simulink model "PropGlycAdjustedARNew1"  (R2019a)
settings: Solver=FixedStepAuto  StartTime=0.0  StopTime=4000  FixedStep=0.1  RelTol=1e-3
values from neighbouring files (symbols this model uses):
  As = pi*r^2    (= 1.89569430983)    [GlycolCSTRparam.m]
  Atank = 6^2*pi()    [GlycolCSTRparam.m]
  Cpa = 35    [GlycolCSTRparam.m]
  Cpb = 18    [GlycolCSTRparam.m]
  Cpc = 46    [GlycolCSTRparam.m]
  Cpm = 19.5    [GlycolCSTRparam.m]
  Cpw = 18    [GlycolCSTRparam.m]
  den = 2.6729    [GlycolCSTRparam.m]
  dh = -36000    [GlycolCSTRparam.m]
  EA = 32400    [GlycolCSTRparam.m]
  Fao = 80    [GlycolCSTRparam.m]
  Fbo = 1000    [GlycolCSTRparam.m]    (also in groundtruth.m)
  Fmo = 100    [GlycolCSTRparam.m]    (also in groundtruth.m)
  htankmax = Vtankmax/Atank    [GlycolCSTRparam.m]
  Hvap = 18279    [GlycolCSTRparam.m]
  Kla = 0    [GlycolCSTRparam.m]
  ko = 16.96e12    (= 16960000000000)    [GlycolCSTRparam.m]
  KT = -10    [GlycolCSTRparam.m]
  Ktank = -1000    [GlycolCSTRparam.m]
  KTank1 = -20    [GlycolCSTRparam.m]
  mc = 1000    [GlycolCSTRparam.m]
  pa = 0.923    [GlycolCSTRparam.m]
  pb = 3.45    [GlycolCSTRparam.m]
  pm = 1.54    [GlycolCSTRparam.m]
  R = 1.987    [GlycolCSTRparam.m]
  RandomMatrix = RandomSetTest    [FinalThesis.m]
  tauT = 2    [GlycolCSTRparam.m]
  tauTank = 0.2    [GlycolCSTRparam.m]
  Tc = 60    [GlycolCSTRparam.m]    (also in groundtruth.m)
  To = 75    [GlycolCSTRparam.m]    (also in groundtruth.m)
  UA = 16000    [GlycolCSTRparam.m]
  V = (1/7.484)*500    (= 66.8091929449)    [GlycolCSTRparam.m]    (also in PCmodel.m = fliplr(V); isstat.m = D(:,j)'; isstatshift.m = D(:,j)')
  Vo = Fao/0.923+Fbo/3.45+Fmo/1.54    (= 441.46402689)    [GlycolCSTRparam.m]
undefined symbols (not defined in the file or in its folder): Tb
settings Model: Creator=19184956  LastModifiedBy=19184956

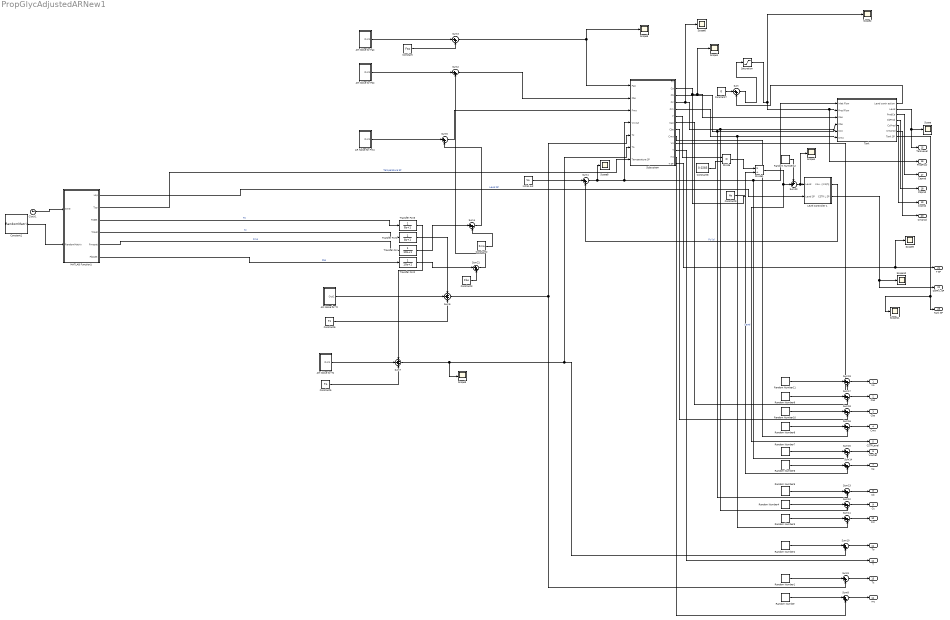
== system PropGlycAdjustedARNew1 ==
  AR Noise for Fao : Subsystem
  AR Noise for Fbo : Subsystem
  AR Noise for Fmo : Subsystem
  AR Noise for Tc : Subsystem
  AR Noise for To : Subsystem
  Clock1 : Clock
  Constant : Constant  Value=Fao
  Constant1 : Constant  Value=RandomMatrix  VectorParams1D=off  SampleTime=-1
  Constant2 : Constant  Value=Fmo
  Constant3 : Constant  Value=Fbo
  Constant5 : Constant  Value=To
  Constant6 : Constant  Value=Tc
  Constant7 : Constant  Value=0
  Constant8 : Constant  Value=0.0283
  Constant9 : Constant  Value=As
  Divide : Product  Inputs=**
  Divide1 : Product  Inputs=*/
  Initial out : Constant  Value=Vo
  Level Controller 1 : Subsystem
  MATLAB Function1 : MATLAB Function  TreatAsAtomicUnit=on
  Random Number{,1..2,7,11} (5 alike) : RandomNumber  Variance=0.5  SampleTime=0.1
  Random Number{3..6,8..10} (7 alike) : RandomNumber  Variance=0.0000025  SampleTime=0.1
  Random Number12 : RandomNumber  Variance=0.0002  SampleTime=0.1
  Saturation : Saturate  UpperLimit=inf  LowerLimit=0
  Scope{,1..6,8..11} (11 alike) : Scope
  Subsystem : Subsystem
  Sum{,1..5,8..19,21} (19 alike) : Sum  Inputs=|++
  Sum20 : Sum  Inputs=++|
  Sum6 : Sum  Inputs=+++
  Sum7 : Sum  Inputs=+++
  Tank : Subsystem
  Transfer Fcn : TransferFcn  Denominator=[10 1]
  Transfer Fcn1 : TransferFcn  Denominator=[8 1]
  Transfer Fcn2 : TransferFcn  Denominator=[10 1]
  Transfer Fcn3 : TransferFcn  Denominator=[8 1]
  Vo : Outport
  Cao : Outport  Port=2
  Cbo : Outport  Port=3
  Cmo : Outport  Port=4
  CSTRLevel : Outport  Port=5
  Voutlet : Outport  Port=6
  Ca : Outport  Port=7
  Cb : Outport  Port=8
  Cc : Outport  Port=9
  Cm : Outport  Port=10
  To : Outport  Port=11
  T : Outport  Port=12
  Tc : Outport  Port=13
  mc : Outport  Port=14
  TankLevel : Outport  Port=15
  ProdFlow : Outport  Port=16
  Caprod : Outport  Port=17
  Cbprod : Outport  Port=18
  Ccprod : Outport  Port=19
  Cmprod : Outport  Port=20
  T SP : Outport  Port=21
  CSTR L SP : Outport  Port=22
  Tank SP : Outport  Port=23
  wires:
  Sum2/1 -> Subsystem/2(Fbo)
  Constant2/1 -> Sum4/2
  Initial out/1 -> Sum1/1
  Sum6/1 -> Subsystem/5(Tc), Sum9/2
  Sum7/1 -> Scope3/1, Sum10/2, Subsystem/6(To)
  Subsystem/2(Ca) -> Sum14/2, Tank/3(Cao), Scope1/1
  Subsystem/3(Cb) -> Tank/4(Cbo), Sum13/2
  Subsystem/4(Cc) -> Scope6/1, Tank/5(Cco), Sum12/2
  Subsystem/5(Cm) -> Tank/6(Cmo), Sum11/2
  Sum/1 -> Saturation/1
  Tank/2(Level) -> TankLevel/1, Scope/1
  Constant7/1 -> Sum/1
  Tank/1(Level contr action) -> Sum/2
  Subsystem/6(V) -> Divide/1
  Constant8/1 -> Divide/2
  Divide/1 -> Divide1/1
  Constant9/1 -> Divide1/2
  Divide1/1 -> CSTRLevel/1, Sum20/2  "Level"
  Level Controller 1/1(Vout'(s) [m3/h]) -> Sum1/2  "Fc'(s)"
  Sum1/1 -> Scope8/1, Tank/1(Inlet Flow), Sum15/2, Subsystem/4(Vo out)
  Saturation/1 -> Scope2/1, ProdFlow/1, Tank/2(Prod Flow)
  Subsystem/10(Vo) -> Sum19/2
  Subsystem/7(Cao) -> Sum17/2
  Subsystem/8(Cbo) -> Sum18/2
  Subsystem/9(Cmo) -> Sum16/2
  Subsystem/11(T) -> T/1
  Subsystem/12(mc) -> Sum8/2
  Tank/3(ProdCa) -> Caprod/1
  Tank/4(CbProd) -> Cbprod/1
  Tank/5(CcProd) -> Ccprod/1
  Tank/6(Cmprod) -> Cmprod/1
  Subsystem/13(T SP) -> Scope9/1, T SP/1
  Level Controller 1/2(CSTR L SP) -> CSTR L SP/1, Scope10/1
  Tank/7("Tank SP ") -> Scope11/1, Tank SP/1
  Sum3/1 -> Subsystem/1(Fao), Scope5/1
  MATLAB Function1/2(Tsp) -> Subsystem/7(Temperature SP)  "Temperature SP"
  MATLAB Function1/1(Lsp) -> Level Controller 1/2(Level SP)  "Level SP"
  Transfer Fcn/1 -> Sum4/1
  Constant/1 -> Sum3/2
  Sum5/1 -> Subsystem/3(Fmo)
  AR Noise for Fao/1(Out1) -> Sum3/1
  AR Noise for Fbo/1(Out1) -> Sum2/1
  Sum4/1 -> Sum5/2
  AR Noise for Fmo/1(Out1) -> Sum5/1
  Constant6/1 -> Sum6/3
  Random Number/1 -> Sum8/1
  Sum8/1 -> mc/1
  Sum9/1 -> Tc/1
  Random Number1/1 -> Sum9/1
  Random Number2/1 -> Sum10/1
  Sum10/1 -> To/1
  Random Number3/1 -> Sum11/1
  Sum11/1 -> Cm/1
  Random Number4/1 -> Sum12/1
  Random Number5/1 -> Sum13/1
  Random Number6/1 -> Sum14/1
  Sum12/1 -> Cc/1
  Sum13/1 -> Cb/1
  Sum14/1 -> Ca/1
  Random Number7/1 -> Sum15/1
  Sum15/1 -> Voutlet/1
  Sum16/1 -> Cmo/1
  Random Number8/1 -> Sum16/1
  Sum17/1 -> Cao/1
  Random Number9/1 -> Sum17/1
  Sum18/1 -> Cbo/1
  Random Number10/1 -> Sum18/1
  Sum19/1 -> Vo/1
  Random Number11/1 -> Sum19/1
  Sum20/1 -> Scope4/1, Level Controller 1/1(Level)
  Random Number12/1 -> Sum20/1
  Transfer Fcn1/1 -> Sum6/1
  AR Noise for Tc/1(Out1) -> Sum6/2
  Transfer Fcn2/1 -> Sum21/1
  Constant3/1 -> Sum21/2
  Sum21/1 -> Sum2/2
  Transfer Fcn3/1 -> Sum7/1
  AR Noise for To/1(Out1) -> Sum7/2
  Constant5/1 -> Sum7/3
  Constant1/1 -> MATLAB Function1/2(RandomMatrix)
  Clock1/1 -> MATLAB Function1/1(time)
  MATLAB Function1/4(Tcset) -> Transfer Fcn1/1  "Tc"
  MATLAB Function1/6(Fboset) -> Transfer Fcn2/1  "Fbo"
  MATLAB Function1/3(ToSet) -> Transfer Fcn3/1  "To"
  MATLAB Function1/5(Fmoset) -> Transfer Fcn/1  "Fmo"

== system PropGlycAdjustedARNew1/AR Noise for Fao ==
  Clock1 : Clock
  Gain : Gain  Gain=0.7
  Random Number : RandomNumber  Variance=0.005  SampleTime=2
  Random Number1 : RandomNumber  Variance=0.005  SampleTime=0.5
  Sum2 : Sum  Inputs=|++
  Switch : Switch  Criteria=u2 > Threshold  Threshold=10
  Transport Delay : TransportDelay  DelayTime=2
  Out1 : Outport
  wires:
  Random Number1/1 -> Switch/3
  Gain/1 -> Sum2/1
  Sum2/1 -> Out1/1, Transport Delay/1
  Random Number/1 -> Switch/1
  Switch/1 -> Sum2/2
  Clock1/1 -> Switch/2
  Transport Delay/1 -> Gain/1

== system PropGlycAdjustedARNew1/AR Noise for Fbo ==
  Clock1 : Clock
  Gain : Gain  Gain=0.7
  Random Number : RandomNumber  Variance=0.005  SampleTime=2
  Random Number1 : RandomNumber  Variance=0.005  SampleTime=0.5
  Scope : Scope
  Sum2 : Sum  Inputs=|++
  Switch : Switch  Criteria=u2 > Threshold  Threshold=10
  Transport Delay : TransportDelay  DelayTime=2
  Out1 : Outport
  wires:
  Random Number1/1 -> Switch/3
  Gain/1 -> Sum2/1
  Sum2/1 -> Scope/1, Out1/1, Transport Delay/1
  Random Number/1 -> Switch/1
  Switch/1 -> Sum2/2
  Clock1/1 -> Switch/2
  Transport Delay/1 -> Gain/1

== system PropGlycAdjustedARNew1/AR Noise for Fmo ==
  Clock1 : Clock
  Gain : Gain  Gain=0.7
  Random Number : RandomNumber  Variance=0.005  SampleTime=2
  Random Number1 : RandomNumber  Variance=0  SampleTime=0.5
  Sum2 : Sum  Inputs=|++
  Switch : Switch  Criteria=u2 > Threshold  Threshold=10
  Transport Delay : TransportDelay  DelayTime=2
  Out1 : Outport
  wires:
  Random Number1/1 -> Switch/3
  Gain/1 -> Sum2/1
  Sum2/1 -> Out1/1, Transport Delay/1
  Random Number/1 -> Switch/1
  Switch/1 -> Sum2/2
  Clock1/1 -> Switch/2
  Transport Delay/1 -> Gain/1

== system PropGlycAdjustedARNew1/AR Noise for Tc ==
  Clock1 : Clock
  Gain : Gain  Gain=0.7
  Random Number : RandomNumber  Variance=0.05  SampleTime=2
  Random Number1 : RandomNumber  Variance=0  SampleTime=0.5
  Sum2 : Sum  Inputs=|++
  Switch : Switch  Criteria=u2 > Threshold  Threshold=10
  Transport Delay : TransportDelay  DelayTime=2
  Out1 : Outport
  wires:
  Random Number1/1 -> Switch/3
  Gain/1 -> Sum2/1
  Sum2/1 -> Out1/1, Transport Delay/1
  Random Number/1 -> Switch/1
  Switch/1 -> Sum2/2
  Clock1/1 -> Switch/2
  Transport Delay/1 -> Gain/1

== system PropGlycAdjustedARNew1/AR Noise for To ==
  Clock1 : Clock
  Gain : Gain  Gain=0.7
  Random Number : RandomNumber  Variance=0.05  SampleTime=2
  Random Number1 : RandomNumber  Variance=0  SampleTime=0.5
  Sum2 : Sum  Inputs=|++
  Switch : Switch  Criteria=u2 > Threshold  Threshold=10
  Transport Delay : TransportDelay  DelayTime=2
  Out1 : Outport
  wires:
  Random Number1/1 -> Switch/3
  Gain/1 -> Sum2/1
  Sum2/1 -> Out1/1, Transport Delay/1
  Random Number/1 -> Switch/1
  Switch/1 -> Sum2/2
  Clock1/1 -> Switch/2
  Transport Delay/1 -> Gain/1

== system PropGlycAdjustedARNew1/Level Controller 1 ==
  Level : Inport
  Level SP : Inport  Port=2
  Constant1 : Constant  Value=0.98
  Gain5 : Gain  Gain=KTank1
  Gc1 : TransferFcn  Numerator=[tauTank 1]  Denominator=[tauTank 0]
  Scope : Scope
  Sum : Sum  Inputs=-+|
  Sum1 : Sum  Inputs=|-+
  Transfer Fcn : TransferFcn  Denominator=[4 1]
  Vout'(s) [m3/h] : Outport
  CSTR L SP : Outport  Port=2
  wires:
  Sum/1 -> Sum1/1  "T'(s)"
  Sum1/1 -> Gain5/1  "E1(s) [K]"
  Constant1/1 -> Sum/1
  Gc1/1 -> Scope/1, Vout'(s) [m3/h]/1  "Vout'(s) [m3/h]"
  Level SP/1 -> Transfer Fcn/1, CSTR L SP/1
  Gain5/1 -> Gc1/1
  Level/1 -> Sum/2
  Transfer Fcn/1 -> Sum1/2

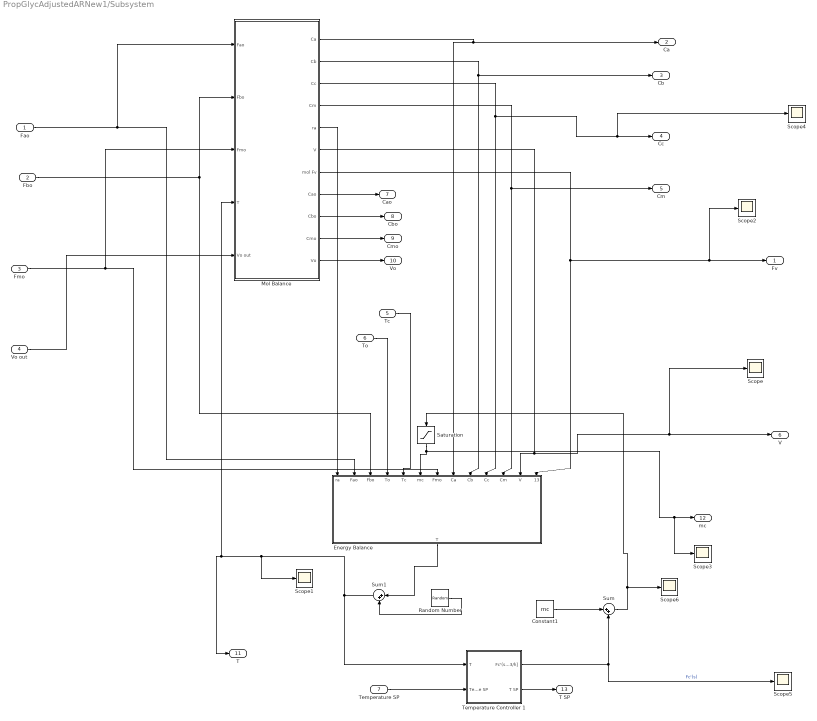
== system PropGlycAdjustedARNew1/Subsystem ==
  Fao : Inport
  Fbo : Inport  Port=2
  Fmo : Inport  Port=3
  Vo out : Inport  Port=4
  Tc : Inport  Port=5
  To : Inport  Port=6
  Temperature SP : Inport  Port=7
  Constant1 : Constant  Value=mc
  Energy Balance : Subsystem
  Mol Balance : Subsystem
  Random Number : RandomNumber  Variance=0.005  SampleTime=0.1
  Saturation : Saturate  UpperLimit=inf  LowerLimit=10
  Scope{,1..6} (7 alike) : Scope
  Sum : Sum  Inputs=|++
  Sum1 : Sum  Inputs=|++
  Temperature Controller 1 : Subsystem
  Fv : Outport
  Ca : Outport  Port=2
  Cb : Outport  Port=3
  Cc : Outport  Port=4
  Cm : Outport  Port=5
  V : Outport  Port=6
  Cao : Outport  Port=7
  Cbo : Outport  Port=8
  Cmo : Outport  Port=9
  Vo : Outport  Port=10
  T : Outport  Port=11
  mc : Outport  Port=12
  T SP : Outport  Port=13
  wires:
  Fmo/1 -> Energy Balance/7(Fmo), Mol Balance/3(Fmo)
  Tc/1 -> Energy Balance/5(Tc)
  Mol Balance/2(Cb) -> Energy Balance/9(Cb), Cb/1
  Mol Balance/4(Cm) -> Cm/1, Energy Balance/11(Cm)
  Mol Balance/7(mol Fv) -> Scope2/1, Fv/1, Energy Balance/13("Fv mol ")
  Mol Balance/3(Cc) -> Scope4/1, Cc/1, Energy Balance/10(Cc)
  Vo out/1 -> Mol Balance/5(Vo out)
  Mol Balance/5(ra) -> Energy Balance/1(ra)
  Fbo/1 -> Energy Balance/3(Fbo), Mol Balance/2(Fbo)
  To/1 -> Energy Balance/4(To)
  Fao/1 -> Energy Balance/2(Fao), Mol Balance/1(Fao)
  Mol Balance/1(Ca) -> Ca/1, Energy Balance/8(Ca)
  Mol Balance/6(V) -> Scope/1, V/1, Energy Balance/12(V)
  Temperature Controller 1/1(Fc'(s) [m3/h]) -> Scope5/1, Sum/2  "Fc'(s)"
  Constant1/1 -> Sum/1
  Sum/1 -> Scope6/1, Saturation/1
  Mol Balance/8(Cao) -> Cao/1
  Mol Balance/9(Cbo) -> Cbo/1
  Mol Balance/10(Cmo) -> Cmo/1
  Mol Balance/11(Vo) -> Vo/1
  Sum1/1 -> Scope1/1, T/1, Mol Balance/4(T), Temperature Controller 1/1(T)
  Temperature Controller 1/2(T SP) -> T SP/1
  Saturation/1 -> Scope3/1, mc/1, Energy Balance/6(mc)
  Temperature SP/1 -> Temperature Controller 1/2(Temperature SP)
  Random Number/1 -> Sum1/2
  Energy Balance/1(T) -> Sum1/1

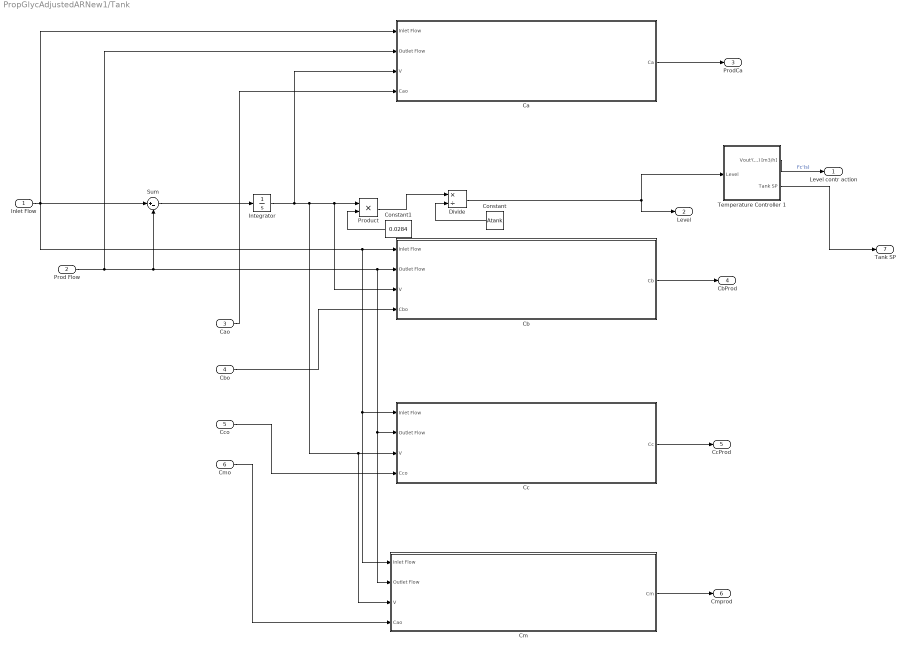
== system PropGlycAdjustedARNew1/Tank ==
  Inlet Flow : Inport
  Prod Flow : Inport  Port=2
  Cao : Inport  Port=3
  Cbo : Inport  Port=4
  Cco : Inport  Port=5
  Cmo : Inport  Port=6
  Ca : Subsystem
  Cb : Subsystem
  Cc : Subsystem
  Cm : Subsystem
  Constant : Constant  Value=Atank
  Constant1 : Constant  Value=0.0284
  Divide : Product  Inputs=*/
  Integrator : Integrator  InitialCondition=V*0.1  UpperSaturationLimit=V
  Product : Product
  Sum : Sum  Inputs=|+-
  Temperature Controller 1 : Subsystem
  Level contr action : Outport
  Level : Outport  Port=2
  ProdCa : Outport  Port=3
  CbProd : Outport  Port=4
  CcProd : Outport  Port=5
  Cmprod : Outport  Port=6
  "Tank SP " : Outport  Port=7
  wires:
  Integrator/1 -> Ca/3(V), Cm/3(V), Cc/3(V), Product/1, Cb/3(V)
  Sum/1 -> Integrator/1
  Inlet Flow/1 -> Ca/1(Inlet Flow), Cm/1(Inlet Flow), Cc/1(Inlet Flow), Cb/1(Inlet Flow), Sum/1
  Prod Flow/1 -> Ca/2(Outlet Flow), Cm/2(Outlet Flow), Cc/2(Outlet Flow), Cb/2(Outlet Flow), Sum/2
  Cao/1 -> Ca/4(Cao)
  Cbo/1 -> Cb/4(Cbo)
  Cco/1 -> Cc/4(Cco)
  Cmo/1 -> Cm/4(Cao)
  Constant/1 -> Divide/2
  Divide/1 -> Temperature Controller 1/1(Level), Level/1
  Temperature Controller 1/1(Vout'(s) [m3/h]) -> Level contr action/1  "Fc'(s)"
  Constant1/1 -> Product/2
  Product/1 -> Divide/1
  Ca/1(Ca) -> ProdCa/1
  Cb/1(Cb) -> CbProd/1
  Cc/1(Cc) -> CcProd/1
  Cm/1(Cm) -> Cmprod/1
  Temperature Controller 1/2(Tank SP) -> "Tank SP "/1

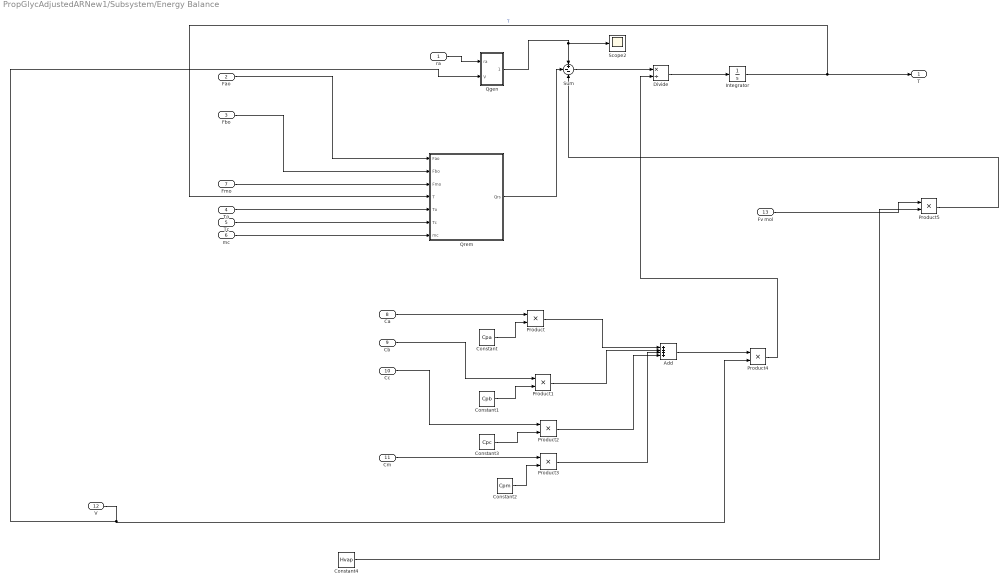
== system PropGlycAdjustedARNew1/Subsystem/Energy Balance ==
  ra : Inport
  Fao : Inport  Port=2
  Fbo : Inport  Port=3
  To : Inport  Port=4
  Tc : Inport  Port=5
  mc : Inport  Port=6
  Fmo : Inport  Port=7
  Ca : Inport  Port=8
  Cb : Inport  Port=9
  Cc : Inport  Port=10
  Cm : Inport  Port=11
  V : Inport  Port=12
  "Fv mol " : Inport  Port=13
  Add : Sum  Inputs=++++
  Constant : Constant  Value=Cpa
  Constant1 : Constant  Value=Cpb
  Constant2 : Constant  Value=Cpm
  Constant3 : Constant  Value=Cpc
  Constant4 : Constant  Value=Hvap
  Divide : Product  Inputs=*/
  Integrator : Integrator  InitialCondition=To  UpperSaturationLimit=Tb+0.5
  Product{,1..5} (6 alike) : Product
  Qgen : Subsystem
  Qrem : Subsystem
  Scope2 : Scope
  Sum : Sum  Inputs=+--
  T : Outport
  wires:
  Integrator/1 -> T/1, Qrem/4(T)  "T"
  ra/1 -> Qgen/1(ra)
  Qrem/1(Qrs) -> Sum/2
  Fao/1 -> Qrem/1(Fao)
  Fbo/1 -> Qrem/2(Fbo)
  To/1 -> Qrem/5(To)
  Tc/1 -> Qrem/6(Tc)
  mc/1 -> Qrem/7(mc)
  Fmo/1 -> Qrem/3(Fmo)
  Ca/1 -> Product/1
  Cb/1 -> Product1/1
  Cc/1 -> Product2/1
  Cm/1 -> Product3/1
  Constant/1 -> Product/2
  Constant1/1 -> Product1/2
  Constant3/1 -> Product2/2
  Constant2/1 -> Product3/2
  Product/1 -> Add/1
  Product1/1 -> Add/2
  Product2/1 -> Add/4
  Product3/1 -> Add/3
  Add/1 -> Product4/1
  V/1 -> Product4/2, Qgen/2(V)
  Product4/1 -> Divide/2
  Constant4/1 -> Product5/2
  Qgen/1(Qgen) -> Sum/1, Scope2/1
  Product5/1 -> Sum/3
  "Fv mol "/1 -> Product5/1
  Sum/1 -> Divide/1
  Divide/1 -> Integrator/1

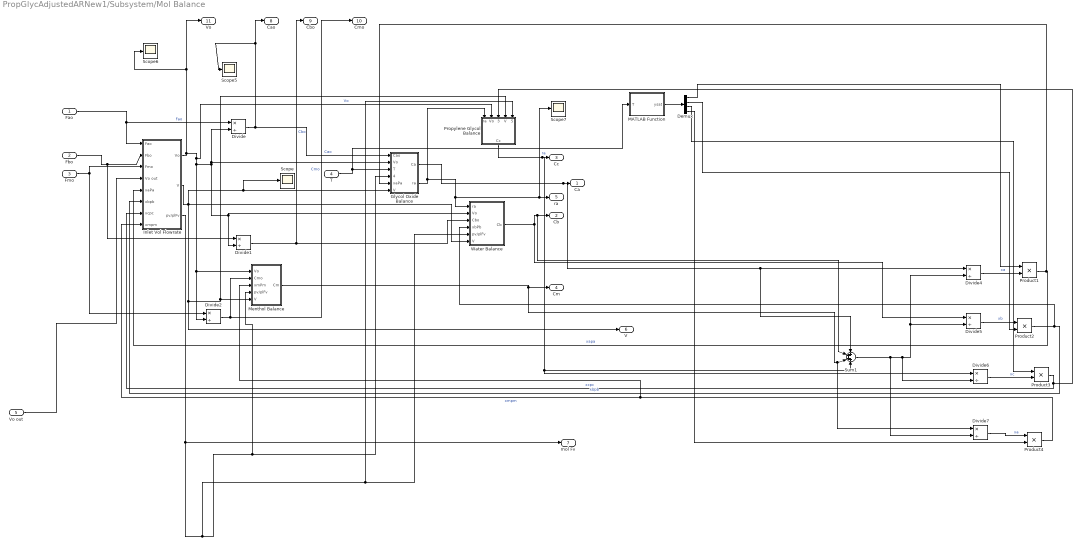
== system PropGlycAdjustedARNew1/Subsystem/Mol Balance ==
  Fao : Inport
  Fbo : Inport  Port=2
  Fmo : Inport  Port=3
  T : Inport  Port=4
  Vo out : Inport  Port=5
  Demux : Demux
  Divide{,1..2,4..7} (7 alike) : Product  Inputs=*/
  Glycol Oxide Balance : Subsystem
  Inlet Vol Flowrate : Subsystem
  MATLAB Function : MATLAB Function  TreatAsAtomicUnit=on
  Menthol Balance : Subsystem
  Product{1..4} (4 alike) : Product
  Propylene Glycol Balance : Subsystem
  Scope{,5..7} (4 alike) : Scope
  Sum1 : Sum  Inputs=++++
  Water Balance : Subsystem
  Ca : Outport
  Cb : Outport  Port=2
  Cc : Outport  Port=3
  Cm : Outport  Port=4
  ra : Outport  Port=5
  V : Outport  Port=6
  mol Fv : Outport  Port=7
  Cao : Outport  Port=8
  Cbo : Outport  Port=9
  Cmo : Outport  Port=10
  Vo : Outport  Port=11
  wires:
  Inlet Vol Flowrate/1(Vo) -> Scope6/1, Vo/1, Propylene Glycol Balance/2(Vo), Divide2/2, Menthol Balance/1(Vo), Divide/2, Glycol Oxide Balance/2(Vo), Divide1/2, Water Balance/2(Vo)  "Vo"
  Fao/1 -> Inlet Vol Flowrate/1(Fao), Divide/1  "Fao"
  Fmo/1 -> Divide2/1, Inlet Vol Flowrate/3(Fmo)
  T/1 -> MATLAB Function/1(T), Glycol Oxide Balance/3(T)
  Fbo/1 -> Divide1/1, Inlet Vol Flowrate/2(Fbo)
  Glycol Oxide Balance/1(Ca) -> Divide4/1, Sum1/1, Ca/1
  Divide/1 -> Glycol Oxide Balance/1(Cao), Cao/1, Scope5/1  "Cao"
  Glycol Oxide Balance/2(ra) -> Propylene Glycol Balance/1(ra), Scope7/1, ra/1, Water Balance/1(ra)  "ra"
  Divide1/1 -> Cbo/1, Water Balance/3(Cbo)  "Cbo"
  Water Balance/1(Cb) -> Sum1/2, Cb/1, Divide5/1
  Divide2/1 -> Cmo/1, Menthol Balance/2(Cmo)  "Cmo"
  Vo out/1 -> Inlet Vol Flowrate/4(Vo out)
  Demux/3 -> Product3/1
  Demux/1 -> Product1/1
  Demux/2 -> Product2/2
  Demux/4 -> Product4/2
  MATLAB Function/1(ysat) -> Demux/1
  Inlet Vol Flowrate/2(V) -> Scope/1, Glycol Oxide Balance/6(V), V/1, Menthol Balance/5(V), Propylene Glycol Balance/4(V), Water Balance/6(V)
  Propylene Glycol Balance/1(Cc) -> Divide6/1, Sum1/4, Cc/1
  Sum1/1 -> Divide7/2, Divide6/2, Divide5/2, Divide4/2
  Divide4/1 -> Product1/2  "xa"
  Product1/1 -> Glycol Oxide Balance/5(xaPa), Inlet Vol Flowrate/5(xaPa)  "xapa"
  Divide5/1 -> Product2/1  "xb"
  Product2/1 -> Water Balance/4(xbPb), Inlet Vol Flowrate/6(xbpb)  "xbpb"
  Divide6/1 -> Product3/2  "xc"
  Product3/1 -> Propylene Glycol Balance/3(xcPc), Inlet Vol Flowrate/7(xcpc)  "xcpc"
  Divide7/1 -> Product4/1  "xa"
  Menthol Balance/1(Cm) -> Divide7/1, Sum1/3, Cm/1
  Product4/1 -> Menthol Balance/3(xmPm), Inlet Vol Flowrate/8(xmpm)  "xmpm"
  Inlet Vol Flowrate/3(pv/plFv) -> Propylene Glycol Balance/5(pv/plFv), Water Balance/5(pv/plFv), Menthol Balance/4(pv/plFv), Glycol Oxide Balance/4(pv/plFv), mol Fv/1

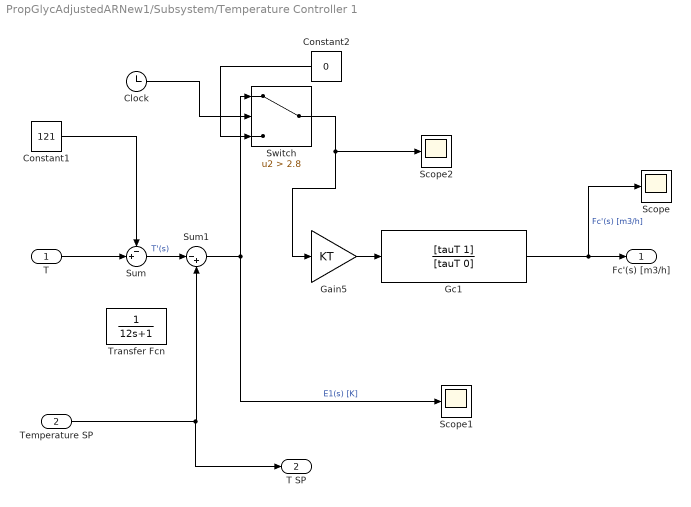
== system PropGlycAdjustedARNew1/Subsystem/Temperature Controller 1 ==
  T : Inport
  Temperature SP : Inport  Port=2
  Clock : Clock
  Constant1 : Constant  Value=121
  Constant2 : Constant  Value=0
  Gain5 : Gain  Gain=KT
  Gc1 : TransferFcn  Numerator=[tauT 1]  Denominator=[tauT 0]
  Scope : Scope
  Scope1 : Scope
  Scope2 : Scope
  Sum : Sum  Inputs=-+|
  Sum1 : Sum  Inputs=|-+
  Switch : Switch  Criteria=u2 > Threshold  Threshold=2.8
  Transfer Fcn : TransferFcn  Denominator=[12 1]
  Fc'(s) [m3/h] : Outport
  T SP : Outport  Port=2
  wires:
  Sum/1 -> Sum1/1  "T'(s)"
  Sum1/1 -> Switch/1, Scope1/1  "E1(s) [K]"
  Constant1/1 -> Sum/1
  Gc1/1 -> Scope/1, Fc'(s) [m3/h]/1  "Fc'(s) [m3/h]"
  Gain5/1 -> Gc1/1
  T/1 -> Sum/2
  Temperature SP/1 -> Sum1/2, T SP/1
  Switch/1 -> Gain5/1, Scope2/1
  Clock/1 -> Switch/2
  Constant2/1 -> Switch/3

== system PropGlycAdjustedARNew1/Tank/Ca ==
  Inlet Flow : Inport
  Outlet Flow : Inport  Port=2
  V : Inport  Port=3
  Cao : Inport  Port=4
  Divide : Product  Inputs=*/
  Integrator : Integrator
  Product : Product
  Product1 : Product
  Sum : Sum  Inputs=|+-
  Ca : Outport
  wires:
  Integrator/1 -> Ca/1, Product1/2
  Sum/1 -> Divide/1
  Inlet Flow/1 -> Product/1
  Cao/1 -> Product/2
  Product/1 -> Sum/1
  Outlet Flow/1 -> Product1/1
  Product1/1 -> Sum/2
  V/1 -> Divide/2
  Divide/1 -> Integrator/1

== system PropGlycAdjustedARNew1/Tank/Cb ==
  Inlet Flow : Inport
  Outlet Flow : Inport  Port=2
  V : Inport  Port=3
  Cbo : Inport  Port=4
  Divide : Product  Inputs=*/
  Integrator : Integrator  InitialCondition=3.45
  Product : Product
  Product1 : Product
  Sum : Sum  Inputs=|+-
  Cb : Outport
  wires:
  Integrator/1 -> Cb/1, Product1/2
  Sum/1 -> Divide/1
  Inlet Flow/1 -> Product/1
  Cbo/1 -> Product/2
  Product/1 -> Sum/1
  Outlet Flow/1 -> Product1/1
  Product1/1 -> Sum/2
  V/1 -> Divide/2
  Divide/1 -> Integrator/1

== system PropGlycAdjustedARNew1/Tank/Cc ==
  Inlet Flow : Inport
  Outlet Flow : Inport  Port=2
  V : Inport  Port=3
  Cco : Inport  Port=4
  Divide : Product  Inputs=*/
  Integrator : Integrator
  Product : Product
  Product1 : Product
  Sum : Sum  Inputs=|+-
  Cc : Outport
  wires:
  Integrator/1 -> Cc/1, Product1/2
  Sum/1 -> Divide/1
  Inlet Flow/1 -> Product/1
  Cco/1 -> Product/2
  Product/1 -> Sum/1
  Outlet Flow/1 -> Product1/1
  Product1/1 -> Sum/2
  V/1 -> Divide/2
  Divide/1 -> Integrator/1

== system PropGlycAdjustedARNew1/Tank/Cm ==
  Inlet Flow : Inport
  Outlet Flow : Inport  Port=2
  V : Inport  Port=3
  Cao : Inport  Port=4
  Divide : Product  Inputs=*/
  Integrator : Integrator
  Product : Product
  Product1 : Product
  Sum : Sum  Inputs=|+-
  Cm : Outport
  wires:
  Integrator/1 -> Cm/1, Product1/2
  Sum/1 -> Divide/1
  Inlet Flow/1 -> Product/1
  Cao/1 -> Product/2
  Product/1 -> Sum/1
  Outlet Flow/1 -> Product1/1
  Product1/1 -> Sum/2
  V/1 -> Divide/2
  Divide/1 -> Integrator/1

== system PropGlycAdjustedARNew1/Tank/Temperature Controller 1 ==
  Level : Inport
  Constant1 : Constant  Value=0
  Gain5 : Gain  Gain=Ktank
  Gc1 : TransferFcn  Numerator=[tauTank 1]  Denominator=[tauTank 0]
  L'sp : Step  Time=0  After=htankmax*0.5  SampleTime=0
  Scope : Scope
  Sum : Sum  Inputs=-+|
  Sum1 : Sum  Inputs=|-+
  Vout'(s) [m3/h] : Outport
  Tank SP : Outport  Port=2
  wires:
  Sum/1 -> Sum1/1  "T'(s)"
  Sum1/1 -> Gain5/1  "E1(s) [K]"
  Constant1/1 -> Sum/1
  Gc1/1 -> Scope/1, Vout'(s) [m3/h]/1  "Vout'(s) [m3/h]"
  L'sp/1 -> Sum1/2, Tank SP/1
  Gain5/1 -> Gc1/1
  Level/1 -> Sum/2

== system PropGlycAdjustedARNew1/Subsystem/Energy Balance/Qgen ==
  ra : Inport
  V : Inport  Port=2
  Constant1 : Constant  Value=dh
  Product : Product  Inputs=3
  Qgen : Outport
  wires:
  ra/1 -> Product/2
  Product/1 -> Qgen/1
  Constant1/1 -> Product/3
  V/1 -> Product/1

== system PropGlycAdjustedARNew1/Subsystem/Energy Balance/Qrem ==
  Fao : Inport
  Fbo : Inport  Port=2
  Fmo : Inport  Port=3
  T : Inport  Port=4
  To : Inport  Port=5
  Tc : Inport  Port=6
  mc : Inport  Port=7
  Qrs1 : Subsystem
  Qrs2 : Subsystem
  Sum1 : Sum  Inputs=|++
  Qrs : Outport
  wires:
  Sum1/1 -> Qrs/1
  Qrs1/1(Qrs1) -> Sum1/1
  Fao/1 -> Qrs1/1(Fao)
  Fbo/1 -> Qrs1/2(Fbo)
  Fmo/1 -> Qrs1/3(Fmo)
  T/1 -> Qrs2/1(T), Qrs1/4(T)
  To/1 -> Qrs1/5(To)
  Qrs2/1(Qrs2) -> Sum1/2
  Tc/1 -> Qrs2/2(Tc)
  mc/1 -> Qrs2/3(mc)

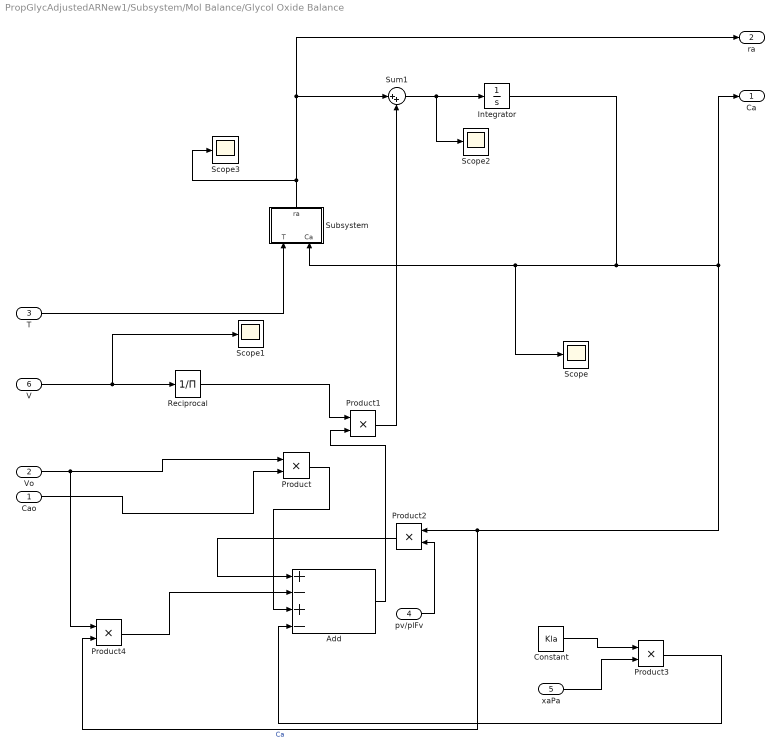
== system PropGlycAdjustedARNew1/Subsystem/Mol Balance/Glycol Oxide Balance ==
  Cao : Inport
  Vo : Inport  Port=2
  T : Inport  Port=3
  pv/plFv : Inport  Port=4
  xaPa : Inport  Port=5
  V : Inport  Port=6
  Add : Sum  Inputs=+-+-
  Constant : Constant  Value=Kla
  Integrator : Integrator  LimitOutput=on  LowerSaturationLimit=0
  Product{,1..4} (5 alike) : Product
  Reciprocal : Product  Inputs=/
  Scope{,1..3} (4 alike) : Scope
  Subsystem : Subsystem
  Sum1 : Sum  Inputs=|++
  Ca : Outport
  ra : Outport  Port=2
  wires:
  Integrator/1 -> Product4/2, Product2/1, Ca/1, Scope/1, Subsystem/2(Ca)  "Ca"
  Cao/1 -> Product/2
  Reciprocal/1 -> Product1/1
  V/1 -> Scope1/1, Reciprocal/1
  Vo/1 -> Product4/1, Product/1
  Sum1/1 -> Scope2/1, Integrator/1
  Product1/1 -> Sum1/2
  T/1 -> Subsystem/1(T)
  Subsystem/1(ra) -> Scope3/1, ra/1, Sum1/1
  Add/1 -> Product1/2
  Product3/1 -> Add/4
  Constant/1 -> Product3/1
  xaPa/1 -> Product3/2
  pv/plFv/1 -> Product2/2
  Product2/1 -> Add/1
  Product/1 -> Add/3
  Product4/1 -> Add/2

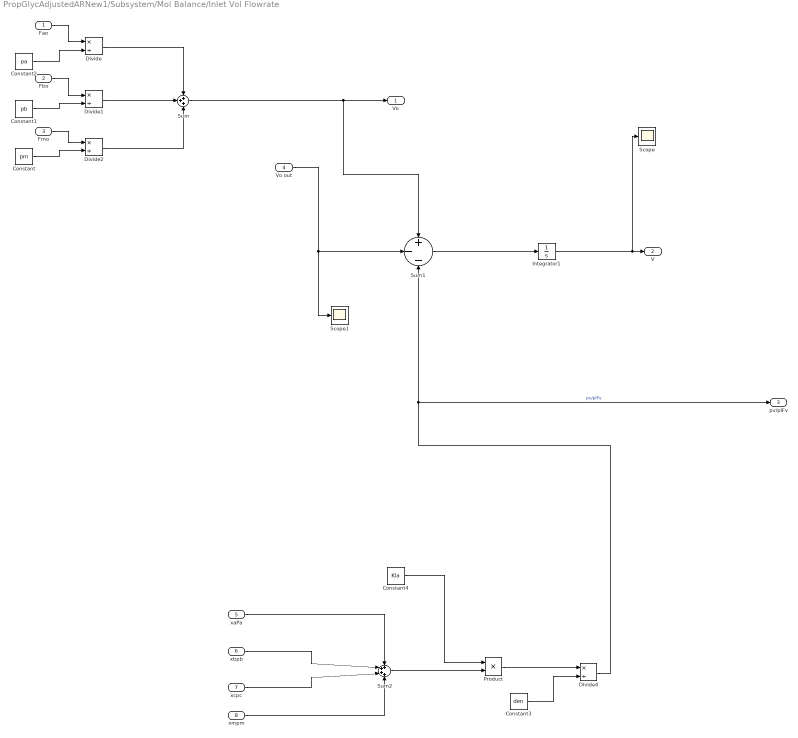
== system PropGlycAdjustedARNew1/Subsystem/Mol Balance/Inlet Vol Flowrate ==
  Fao : Inport
  Fbo : Inport  Port=2
  Fmo : Inport  Port=3
  Vo out : Inport  Port=4
  xaPa : Inport  Port=5
  xbpb : Inport  Port=6
  xcpc : Inport  Port=7
  xmpm : Inport  Port=8
  Constant : Constant  Value=pm
  Constant1 : Constant  Value=pb
  Constant2 : Constant  Value=pa
  Constant3 : Constant  Value=den
  Constant4 : Constant  Value=Kla
  Divide{,1..2,4} (4 alike) : Product  Inputs=*/
  Integrator1 : Integrator  InitialCondition=V  LimitOutput=on  UpperSaturationLimit=V*3  LowerSaturationLimit=0
  Product : Product
  Scope : Scope
  Scope1 : Scope
  Sum : Sum  Inputs=+++
  Sum1 : Sum  Inputs=+--
  Sum2 : Sum  Inputs=++++
  Vo : Outport
  V : Outport  Port=2
  pv/plFv : Outport  Port=3
  wires:
  Divide/1 -> Sum/1
  Constant1/1 -> Divide1/2
  Constant2/1 -> Divide/2
  Divide1/1 -> Sum/2
  Fao/1 -> Divide/1
  Fbo/1 -> Divide1/1
  Divide2/1 -> Sum/3
  Constant/1 -> Divide2/2
  Fmo/1 -> Divide2/1
  Sum/1 -> Sum1/1, Vo/1
  Vo out/1 -> Sum1/2, Scope1/1
  Integrator1/1 -> Scope/1, V/1
  Sum1/1 -> Integrator1/1
  xaPa/1 -> Sum2/1
  xbpb/1 -> Sum2/2
  xcpc/1 -> Sum2/3
  xmpm/1 -> Sum2/4
  Sum2/1 -> Product/2
  Constant4/1 -> Product/1
  Product/1 -> Divide4/1
  Constant3/1 -> Divide4/2
  Divide4/1 -> Sum1/3, pv/plFv/1  "pv/plFv"

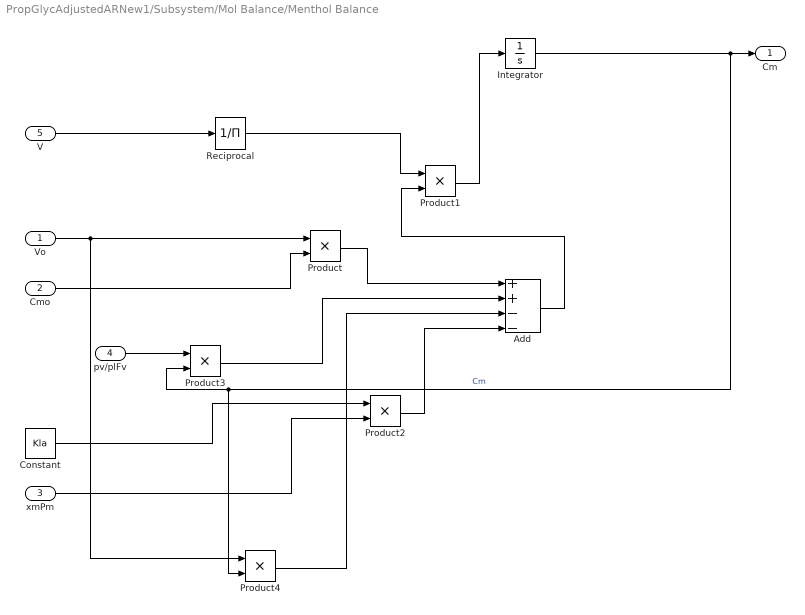
== system PropGlycAdjustedARNew1/Subsystem/Mol Balance/Menthol Balance ==
  Vo : Inport
  Cmo : Inport  Port=2
  xmPm : Inport  Port=3
  pv/plFv : Inport  Port=4
  V : Inport  Port=5
  Add : Sum  Inputs=++--
  Constant : Constant  Value=Kla
  Integrator : Integrator
  Product{,1..4} (5 alike) : Product
  Reciprocal : Product  Inputs=/
  Cm : Outport
  wires:
  Integrator/1 -> Product4/2, Product3/2, Cm/1  "Cm"
  Cmo/1 -> Product/2
  Reciprocal/1 -> Product1/1
  V/1 -> Reciprocal/1
  Vo/1 -> Product4/1, Product/1
  Product/1 -> Add/1
  Product1/1 -> Integrator/1
  Constant/1 -> Product2/1
  xmPm/1 -> Product2/2
  Product2/1 -> Add/4
  Add/1 -> Product1/2
  pv/plFv/1 -> Product3/1
  Product3/1 -> Add/2
  Product4/1 -> Add/3

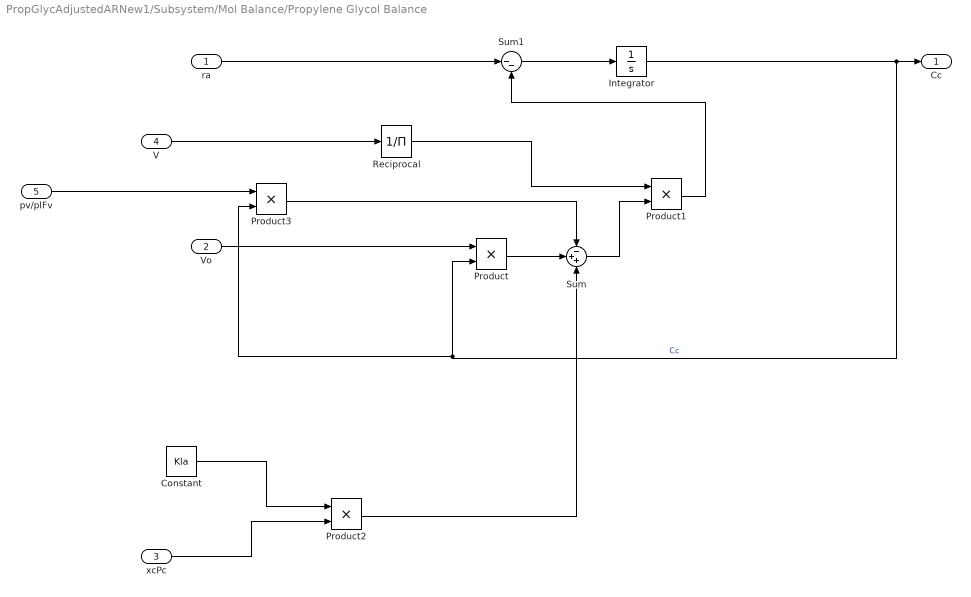
== system PropGlycAdjustedARNew1/Subsystem/Mol Balance/Propylene Glycol Balance ==
  ra : Inport
  Vo : Inport  Port=2
  xcPc : Inport  Port=3
  V : Inport  Port=4
  pv/plFv : Inport  Port=5
  Constant : Constant  Value=Kla
  Integrator : Integrator
  Product{,1..3} (4 alike) : Product
  Reciprocal : Product  Inputs=/
  Sum : Sum  Inputs=-++
  Sum1 : Sum  Inputs=|--
  Cc : Outport
  wires:
  Integrator/1 -> Product3/2, Product/2, Cc/1  "Cc"
  Reciprocal/1 -> Product1/1
  Sum1/1 -> Integrator/1
  Product1/1 -> Sum1/2
  ra/1 -> Sum1/1
  Constant/1 -> Product2/1
  xcPc/1 -> Product2/2
  V/1 -> Reciprocal/1
  Product2/1 -> Sum/3
  Sum/1 -> Product1/2
  Vo/1 -> Product/1
  Product/1 -> Sum/2
  Product3/1 -> Sum/1
  pv/plFv/1 -> Product3/1

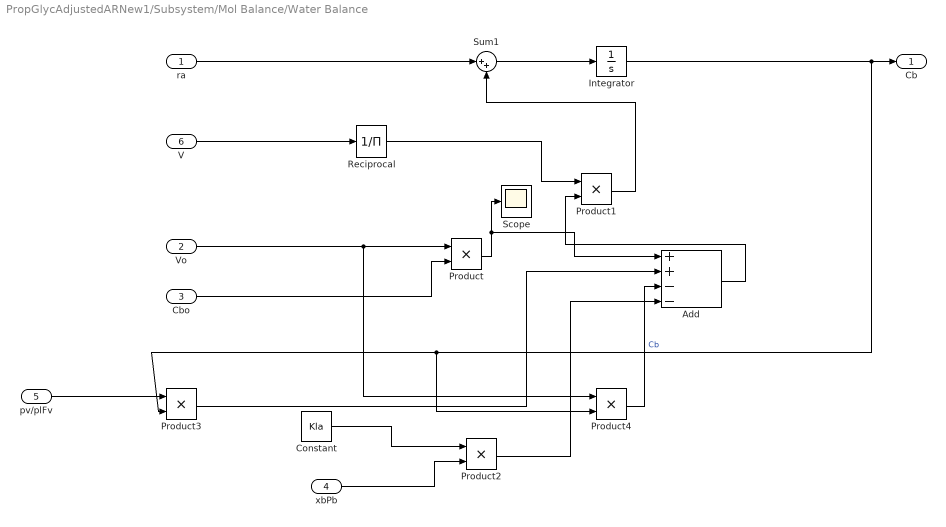
== system PropGlycAdjustedARNew1/Subsystem/Mol Balance/Water Balance ==
  ra : Inport
  Vo : Inport  Port=2
  Cbo : Inport  Port=3
  xbPb : Inport  Port=4
  pv/plFv : Inport  Port=5
  V : Inport  Port=6
  Add : Sum  Inputs=++--
  Constant : Constant  Value=Kla
  Integrator : Integrator  InitialCondition=3.45
  Product{,1..4} (5 alike) : Product
  Reciprocal : Product  Inputs=/
  Scope : Scope
  Sum1 : Sum  Inputs=|++
  Cb : Outport
  wires:
  Integrator/1 -> Product4/2, Product3/2, Cb/1  "Cb"
  Cbo/1 -> Product/2
  Reciprocal/1 -> Product1/1
  V/1 -> Reciprocal/1
  Vo/1 -> Product4/1, Product/1
  Product/1 -> Add/1, Scope/1
  Sum1/1 -> Integrator/1
  Product1/1 -> Sum1/2
  ra/1 -> Sum1/1
  Constant/1 -> Product2/1
  xbPb/1 -> Product2/2
  Product2/1 -> Add/4
  Add/1 -> Product1/2
  pv/plFv/1 -> Product3/1
  Product3/1 -> Add/2
  Product4/1 -> Add/3

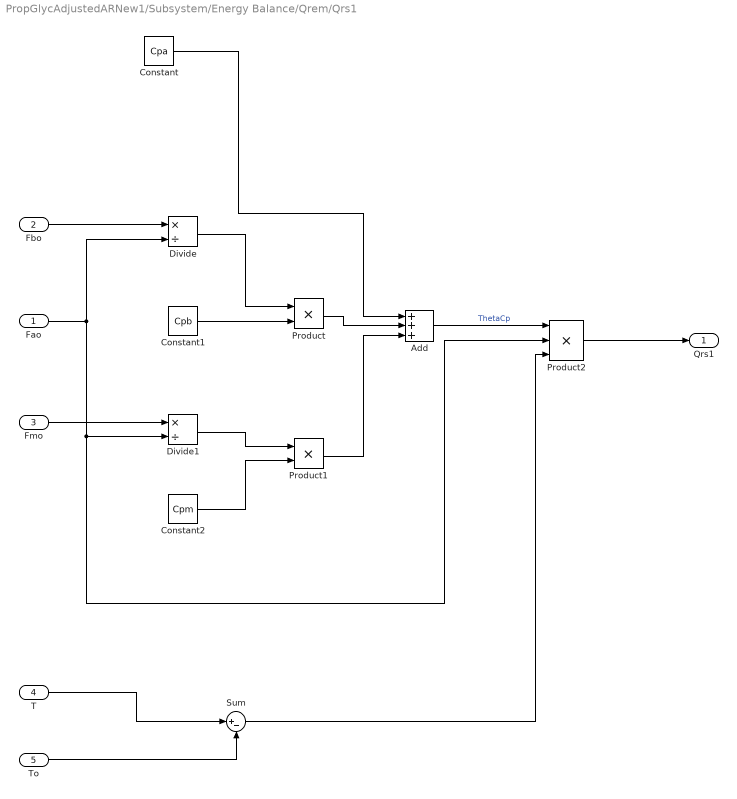
== system PropGlycAdjustedARNew1/Subsystem/Energy Balance/Qrem/Qrs1 ==
  Fao : Inport
  Fbo : Inport  Port=2
  Fmo : Inport  Port=3
  T : Inport  Port=4
  To : Inport  Port=5
  Add : Sum  Inputs=+++
  Constant : Constant  Value=Cpa
  Constant1 : Constant  Value=Cpb
  Constant2 : Constant  Value=Cpm
  Divide : Product  Inputs=*/
  Divide1 : Product  Inputs=*/
  Product : Product
  Product1 : Product
  Product2 : Product  Inputs=3
  Sum : Sum  Inputs=|+-
  Qrs1 : Outport
  wires:
  Sum/1 -> Product2/3
  Constant/1 -> Add/1
  Fao/1 -> Divide/2, Divide1/2, Product2/2
  Fbo/1 -> Divide/1
  Constant1/1 -> Product/2
  Divide/1 -> Product/1
  Fmo/1 -> Divide1/1
  Constant2/1 -> Product1/2
  Divide1/1 -> Product1/1
  Product1/1 -> Add/3
  Product/1 -> Add/2
  Add/1 -> Product2/1  "ThetaCp"
  T/1 -> Sum/1
  To/1 -> Sum/2
  Product2/1 -> Qrs1/1

== system PropGlycAdjustedARNew1/Subsystem/Energy Balance/Qrem/Qrs2 ==
  T : Inport
  Tc : Inport  Port=2
  mc : Inport  Port=3
  Constant : Constant  Value=-1*UA
  Constant1 : Constant  Value=Cpw
  Divide : Product  Inputs=*//
  Exp : Math  SaturateOnIntegerOverflow=on
  Product : Product
  Product1 : Product  Inputs=3
  Scope : Scope
  Scope1 : Scope
  Sum : Sum  Inputs=|+-
  Sum1 : Sum  Inputs=|+-
  Sum2 : Sum  Inputs=+-|
  Qrs2 : Outport
  wires:
  Sum/1 -> Product1/1
  Tc/1 -> Scope1/1, Sum/2, Sum2/2
  T/1 -> Sum2/1, Sum1/1
  Sum2/1 -> Product/1
  Exp/1 -> Product/2
  mc/1 -> Product1/2, Divide/2
  Divide/1 -> Exp/1
  Constant/1 -> Divide/1
  Constant1/1 -> Product1/3, Divide/3
  Product/1 -> Sum1/2
  Sum1/1 -> Scope/1, Sum/1  "Ta2"
  Product1/1 -> Qrs2/1

== system PropGlycAdjustedARNew1/Subsystem/Mol Balance/Glycol Oxide Balance/Subsystem ==
  T : Inport
  Ca : Inport  Port=2
  Constant1 : Constant  Value=-1*ko
  Constant2 : Constant  Value=R
  Constant3 : Constant  Value=0
  Constant4 : Constant  Value=460
  Constant5 : Constant  Value=-1*EA
  Divide : Product  Inputs=//*
  Exp : Math  SaturateOnIntegerOverflow=on
  Product2 : Product
  Product4 : Product
  Scope : Scope
  Scope1 : Scope
  Sum3 : Sum  Inputs=+++
  ra : Outport
  wires:
  Constant5/1 -> Divide/3
  Constant1/1 -> Product2/1
  Constant3/1 -> Sum3/1
  T/1 -> Sum3/2
  Product4/1 -> Scope1/1, ra/1
  Constant4/1 -> Sum3/3
  Exp/1 -> Product2/2
  Product2/1 -> Scope/1, Product4/1
  Constant2/1 -> Divide/1
  Divide/1 -> Exp/1
  Ca/1 -> Product4/2
  Sum3/1 -> Divide/2

== matlab function PropGlycAdjustedARNew1/Subsystem/Mol Balance/MATLAB Function ==
  data: T input; ysat output
function ysat = detSaty(T)
T = (T-32)/(9/5)+273;
Aparamc = [6.079 2692.18 -17.14];
Aparamb = [3.559 643.748 -198.043];
Aparama = [3.55 802.4 -81.34];
Aparamm = [5.1569 1569.6 -34.84];
Patm = 1;

yasat = 10^(Aparama(1)-Aparama(2)/(T+Aparama(3)));
ybsat = 10^(Aparamb(1)-Aparamb(2)/(T+Aparamb(3)));
ycsat = 10^(Aparamc(1)-Aparamc(2)/(T+Aparamc(3)));
ymsat = 10^(Aparamm(1)-Aparamm(2)/(T+Aparamm(3)));

ysat = [yasat ybsat ycsat ymsat];

== matlab function PropGlycAdjustedARNew1/MATLAB Function1 ==
  data: time input; Lsp output; RandomMatrix input; Tsp output; ToSet output; Tcset output; Fmoset output; Fboset output
function [Lsp,Tsp,ToSet,Tcset,Fmoset,Fboset] = fcn(time,RandomMatrix)
RandomMatrix(:,end) = RandomMatrix(:,end)*0.1;
In =  RandomMatrix(RandomMatrix(:,end)>=time,:);
idx = size(In);
if idx ~= size(RandomMatrix,1)
In = RandomMatrix(size(RandomMatrix,1)-idx,:);
end
if time<RandomMatrix(2,end)
    Lsp = 0;
    Tsp = 0;
    ToSet = 0;
    Tcset = 0;
    Fmoset = 0;
    Fboset = 0;
else
    if time>=RandomMatrix(end,end)
        Lsp = RandomMatrix(end,1);
        Tsp = RandomMatrix(end,2);
        ToSet = RandomMatrix(end,3);
        Tcset = RandomMatrix(end,4);
        Fmoset = RandomMatrix(end,5);
        Fboset = RandomMatrix(end,6);
    else
        Lsp = In(1,1);
        Tsp = In(1,2);
        ToSet = In(1,3);
        Tcset = In(1,4);
        Fmoset = In(1,5);
        Fboset = In(1,6);
    end
end
% RandomMatrix(:,end) = RandomMatrix(:,end)*0.1;
% In =  RandomMatrix(RandomMatrix(:,end)>=time,:);
% if time<RandomMatrix(2,end)
%     Lsp = 0;
%     Tsp = 0;
%     ToSet = 0;
%     Tcset = 0;
%     Fmoset = 0;
%     Fboset = 0;
% else
%     if time>=RandomMatrix(end,end)
%         Lsp = RandomMatrix(end,1);
%         Tsp = RandomMatrix(end,2);
%         ToSet = RandomMatrix(end,3);
%         Tcset = RandomMatrix(end,4);
%         Fmoset = RandomMatrix(end,5);
%         Fboset = RandomMatrix(end,6);
%     else
%         Lsp = In(1,1);
%         Tsp = In(1,2);
%         ToSet = In(1,3);
%         Tcset = In(1,4);
%         Fmoset = In(1,5);
%         Fboset = In(1,6);
%     end
% end
